simulink model "half_adder"  (R2021a)
settings: Solver=VariableStepAuto  StartTime=0.0  StopTime=10.0  RelTol=1e-3
settings Model: Creator=kbhar  LastModifiedBy=kbhar

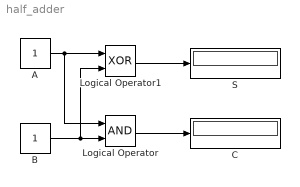
== system half_adder ==
  A : Constant
  B : Constant
  C : Display
  Logical Operator : Logic  AllPortsSameDT=off  OutDataTypeStr=boolean
  Logical Operator1 : Logic  Operator=XOR  AllPortsSameDT=off  OutDataTypeStr=boolean
  S : Display
  wires:
  B/1 -> Logical Operator1/2, Logical Operator/2
  A/1 -> Logical Operator/1, Logical Operator1/1
  Logical Operator/1 -> C/1
  Logical Operator1/1 -> S/1
